simulink model "ABS_CHO"  (R2023a)
settings: Solver=ode45  StartTime=0  StopTime=15  FixedStep=0.001  RelTol=1e-3  AbsTol=1e-6
libraries: simulink x19, dspsigops x7, Solver_SF x1
(part 2 of 2)

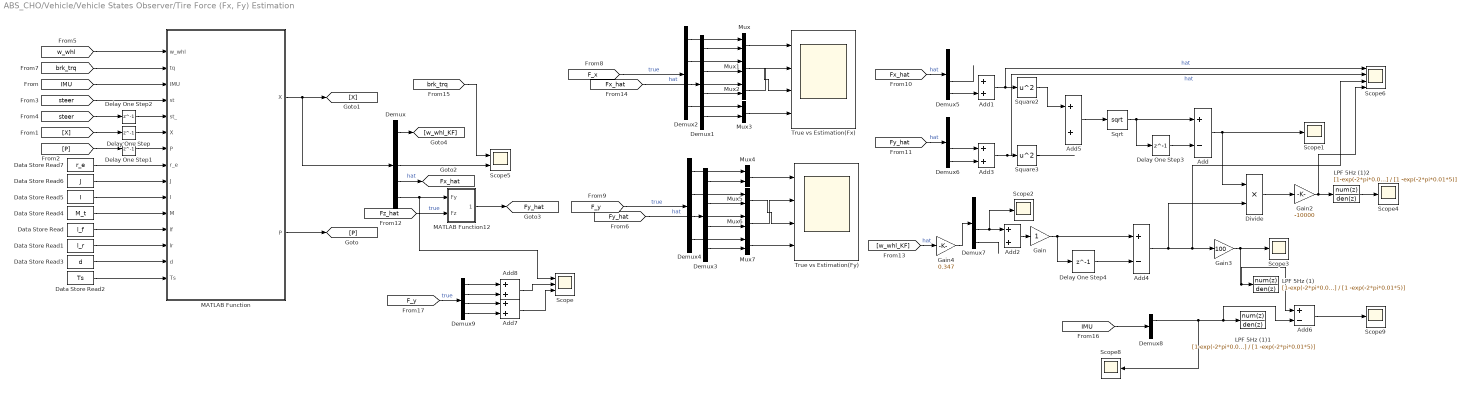
== system ABS_CHO/Vehicle/Vehicle States Observer/Tire Force (Fx, Fy) Estimation ==
  Add : Sum  Inputs=+-
  Add{1..3,5,7..8} (6 alike) : Sum
  Add4 : Sum  Inputs=+-
  Add6 : Sum  Inputs=+-
  Data Store Read : DataStoreRead  DataStoreName=l_f  IndexOptions=Index vector (dialog)  Indices=1  OutputSizes=1
  Data Store Read1 : DataStoreRead  DataStoreName=l_r  IndexOptions=Index vector (dialog)  Indices=1  OutputSizes=1
  Data Store Read2 : DataStoreRead  DataStoreName=Ts  IndexOptions=Index vector (dialog)  Indices=1  OutputSizes=1
  Data Store Read3 : DataStoreRead  DataStoreName=d  IndexOptions=Index vector (dialog)  Indices=1  OutputSizes=1
  Data Store Read4 : DataStoreRead  DataStoreName=M_t  IndexOptions=Index vector (dialog)  Indices=1  OutputSizes=1
  Data Store Read5 : DataStoreRead  DataStoreName=I  IndexOptions=Index vector (dialog)  Indices=1  OutputSizes=1
  Data Store Read6 : DataStoreRead  DataStoreName=J  IndexOptions=Index vector (dialog)  Indices=1  OutputSizes=1
  Data Store Read7 : DataStoreRead  DataStoreName=r_e  IndexOptions=Index vector (dialog)  Indices=1  OutputSizes=1
  Delay One Step : Delay  DelayLength=1  InitialCondition=[80 80 80 80 0 0 0 0 0 0 0 0]'  SampleTime=0.01
  Delay One Step1 : Delay  DelayLength=1  InitialCondition=diag([80 80 80 80 0 0 0 0 0 0 0 0])  SampleTime=0.01
  Delay One Step2 : Delay  DelayLength=1  InitialCondition=[0 0 0 0]'  SampleTime=0.01
  Delay One Step3 : Delay  DelayLength=1
  Delay One Step4 : Delay  DelayLength=1  InitialCondition=27.78
  Demux : Demux  Outputs=[4 1 1 4 2]
  Demux{1..7,9} (8 alike) : Demux
  Demux8 : Demux  Outputs=3
  Divide : Product  Inputs=**
  Gain : Gain
  Gain2 : Gain  Gain=-10000
  Gain3 : Gain  Gain=100
  Gain4 : Gain  Gain=0.347
  LPF 5Hz (1) : DiscreteFilter  Numerator=[1-exp(-2*pi*0.01*5)]  Denominator=[1 -exp(-2*pi*0.01*5)]  SampleTime=0.01
  LPF 5Hz (1)1 : DiscreteFilter  Numerator=[1-exp(-2*pi*0.01*5)]  Denominator=[1 -exp(-2*pi*0.01*5)]  SampleTime=0.01
  LPF 5Hz (1)2 : DiscreteFilter  Numerator=[1-exp(-2*pi*0.01*5)]  Denominator=[1 -exp(-2*pi*0.01*5)]  SampleTime=0.01
  MATLAB Function : MATLAB Function  TreatAsAtomicUnit=on
  MATLAB Function12 : MATLAB Function  TreatAsAtomicUnit=on
  Mux{,1..7} (8 alike) : Mux  Inputs=2
  Scope : Scope  NumInputPorts=3
  Scope{1..4,8..9} (6 alike) : Scope
  Scope5 : Scope  NumInputPorts=2
  Scope6 : Scope  NumInputPorts=4
  Sqrt : Sqrt
  Square2 : Math  Operator=square
  Square3 : Math  Operator=square
  True vs Estimation(Fx) : Scope  NumInputPorts=4
  True vs Estimation(Fy) : Scope  NumInputPorts=4
  tag scope: Fx_hat=global, Fy_hat=global
  wires:
  Data Store Read/1 -> MATLAB Function/12(lf)
  Data Store Read1/1 -> MATLAB Function/13(lr)
  Data Store Read2/1 -> MATLAB Function/15(Ts)
  Data Store Read3/1 -> MATLAB Function/14(d)
  Data Store Read4/1 -> MATLAB Function/11(M)
  Data Store Read5/1 -> MATLAB Function/10(I)
  Data Store Read6/1 -> MATLAB Function/9(J)
  Data Store Read7/1 -> MATLAB Function/8(r_e)
  MATLAB Function/2(P) -> [P]
  MATLAB Function/1(X) -> Demux/1, [X]
  [X] -> Delay One Step/1
  Delay One Step/1 -> MATLAB Function/6("X ")
  [P] -> Delay One Step1/1
  Delay One Step1/1 -> MATLAB Function/7("P ")
  [steer] -> MATLAB Function/4(st)
  [steer] -> Delay One Step2/1
  Delay One Step2/1 -> MATLAB Function/5(st_)
  [w_whl] -> MATLAB Function/1(w_whl)
  Mux2/1 -> True vs Estimation(Fx)/2
  Mux3/1 -> True vs Estimation(Fx)/4
  Demux1/3 -> Mux2/2
  Mux/1 -> True vs Estimation(Fx)/1
  [Fx_hat] -> Demux1/1  "hat"
  Demux1/4 -> Mux3/2
  Demux2/4 -> Mux3/1
  Demux1/2 -> Mux1/2
  Demux1/1 -> Mux/2
  Demux2/1 -> Mux/1
  Demux2/3 -> Mux2/1
  Mux1/1 -> True vs Estimation(Fx)/3
  Demux2/2 -> Mux1/1
  [F_x] -> Demux2/1  "true"
  [IMU] -> MATLAB Function/3(IMU)
  [brk_trq] -> MATLAB Function/2(tq)
  [Fz_hat] -> MATLAB Function12/2(Fz)  "true"
  Demux/4 -> [Fx_hat]  "hat"
  Demux/5 -> Scope/1, MATLAB Function12/1(Fy)
  MATLAB Function12/1(Fyhat) -> [Fy_hat]
  Demux4/1 -> Mux4/1
  Demux4/2 -> Mux5/1
  Demux3/4 -> Mux7/2
  Demux3/2 -> Mux5/2
  Demux3/1 -> Mux4/2
  Demux4/3 -> Mux6/1
  Demux4/4 -> Mux7/1
  Mux7/1 -> True vs Estimation(Fy)/4
  Mux6/1 -> True vs Estimation(Fy)/2
  Demux3/3 -> Mux6/2
  [F_y] -> Demux4/1  "true"
  Mux5/1 -> True vs Estimation(Fy)/3
  Mux4/1 -> True vs Estimation(Fy)/1
  [Fy_hat] -> Demux3/1  "hat"
  [Fx_hat] -> Demux5/1  "hat"
  Add1/1 -> Scope6/1, Square2/1  "hat"
  Demux5/3 -> ?
  Demux5/4 -> Add1/2
  Demux6/3 -> Add3/1
  [Fy_hat] -> Demux6/1  "hat"
  Add3/1 -> Scope6/2, Square3/1  "hat"
  Demux6/4 -> Add3/2
  Square2/1 -> Add5/1
  Square3/1 -> ?
  Delay One Step3/1 -> Add/2
  Add/1 -> Divide/1, Scope1/1
  Add5/1 -> Sqrt/1
  Sqrt/1 -> Delay One Step3/1, Add/1
  [w_whl_KF] -> Gain4/1  "hat"
  Demux7/3 -> Scope2/1, Add2/1
  Demux7/4 -> ?
  Add2/1 -> Gain/1
  Gain/1 -> Delay One Step4/1, Add4/1
  Delay One Step4/1 -> Add4/2
  Add4/1 -> Divide/2, Gain3/1, Scope6/3
  Divide/1 -> Gain2/1
  Demux/3 -> Scope5/2
  [brk_trq] -> Scope5/1
  Gain3/1 -> Add6/1, LPF 5Hz (1)/1, Scope3/1
  Demux/1 -> [w_whl_KF]
  [IMU] -> Demux8/1
  Demux8/1 -> Scope8/1, Add6/2, LPF 5Hz (1)1/1
  Add6/1 -> Scope9/1
  Gain2/1 -> LPF 5Hz (1)2/1, Scope6/4
  LPF 5Hz (1)2/1 -> Scope4/1
  Gain4/1 -> Demux7/1
  [F_y] -> Demux9/1  "true"
  Demux9/4 -> Add7/2
  Demux9/3 -> Add7/1
  Demux9/1 -> Add8/1
  Demux9/2 -> Add8/2
  Add8/1 -> Scope/2
  Add7/1 -> Scope/3

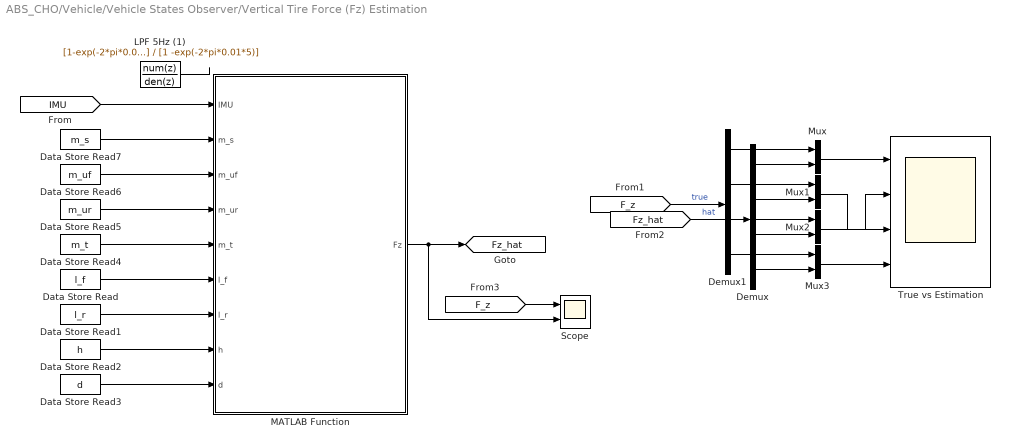
== system ABS_CHO/Vehicle/Vehicle States Observer/Vertical Tire Force (Fz) Estimation ==
  Data Store Read : DataStoreRead  DataStoreName=l_f  IndexOptions=Index vector (dialog)  Indices=1  OutputSizes=1
  Data Store Read1 : DataStoreRead  DataStoreName=l_r  IndexOptions=Index vector (dialog)  Indices=1  OutputSizes=1
  Data Store Read2 : DataStoreRead  DataStoreName=h  IndexOptions=Index vector (dialog)  Indices=1  OutputSizes=1
  Data Store Read3 : DataStoreRead  DataStoreName=d  IndexOptions=Index vector (dialog)  Indices=1  OutputSizes=1
  Data Store Read4 : DataStoreRead  DataStoreName=m_t  IndexOptions=Index vector (dialog)  Indices=1  OutputSizes=1
  Data Store Read5 : DataStoreRead  DataStoreName=m_ur  IndexOptions=Index vector (dialog)  Indices=1  OutputSizes=1
  Data Store Read6 : DataStoreRead  DataStoreName=m_uf  IndexOptions=Index vector (dialog)  Indices=1  OutputSizes=1
  Data Store Read7 : DataStoreRead  DataStoreName=m_s  IndexOptions=Index vector (dialog)  Indices=1  OutputSizes=1
  Demux : Demux
  Demux1 : Demux
  LPF 5Hz (1) : DiscreteFilter  Numerator=[1-exp(-2*pi*0.01*5)]  Denominator=[1 -exp(-2*pi*0.01*5)]  SampleTime=0.01
  MATLAB Function : MATLAB Function  TreatAsAtomicUnit=on
  Mux{,1..3} (4 alike) : Mux  Inputs=2
  Scope : Scope  NumInputPorts=2
  True vs Estimation : Scope  NumInputPorts=4
  tag scope: Fz_hat=global
  wires:
  Data Store Read/1 -> MATLAB Function/6(l_f)
  Data Store Read1/1 -> MATLAB Function/7(l_r)
  Data Store Read2/1 -> MATLAB Function/8(h)
  Data Store Read3/1 -> MATLAB Function/9(d)
  Data Store Read4/1 -> MATLAB Function/5(m_t)
  Data Store Read5/1 -> MATLAB Function/4(m_ur)
  Data Store Read6/1 -> MATLAB Function/3(m_uf)
  Data Store Read7/1 -> MATLAB Function/2(m_s)
  [IMU] -> MATLAB Function/1(IMU)
  MATLAB Function/1(Fz) -> Scope/2, [Fz_hat]
  [F_z] -> Scope/1
  [Fz_hat] -> Demux/1  "hat"
  [F_z] -> Demux1/1  "true"
  Demux1/1 -> Mux/1
  Demux/1 -> Mux/2
  Demux1/2 -> Mux1/1
  Demux/2 -> Mux1/2
  Demux1/3 -> Mux2/1
  Demux/3 -> Mux2/2
  Demux1/4 -> Mux3/1
  Demux/4 -> Mux3/2
  Mux/1 -> True vs Estimation/1
  Mux1/1 -> True vs Estimation/3
  Mux3/1 -> True vs Estimation/4
  Mux2/1 -> True vs Estimation/2
  LPF 5Hz (1)/1 -> ?

== stateflow chart ABS_CHO/ABS_FR/Chart ==
  state ABS_On
    state Phase1
      entry,during:
      phase = 1;
    state Phase2
      entry,during:
      phase = 2;
    state Phase3
      entry,during:
      phase = 3;
    state Phase4
      entry,during:
      phase = 4;
    state Phase5
      entry,during:
      phase = 5;
    state Phase6
      entry,during:
      phase = 6;
    state Phase7
      entry,during:
      phase = 7;
    state Phase8
      entry,during:
      phase = 8;
    (default) -> Phase1
    Phase1 -> Phase2 : [(a_whl<a_whl_thrs1)]
    Phase2 -> Phase3 : [(v_whl<v_whl_thrs)]
    Phase3 -> Phase4 : [(a_whl>a_whl_thrs1)]
    (junction 81) -> Phase4
    (junction 79) -> (junction 81)
    Phase4 -> Phase5 : [(a_whl>a_whl_thrs2)]
    Phase5 -> Phase6 : [(a_whl<a_whl_thrs2)]
    Phase6 -> Phase7 : [(a_whl<a_whl_thrs3)]
    Phase7 -> Phase8 : [(a_whl<a_whl_thrs1)]
    Phase8 -> (junction 79) : [(a_whl>a_whl_thrs1)]
  state ABS_Off
    phase = 0;
  (default) -> ABS_Off
  ABS_Off -> ABS_On : [(P_cmd > P_cmd_min)&(v_car > 2)]
  (junction 96) -> ABS_Off
  ABS_On -> (junction 96) : [(P_cmd < P_cmd_min)|(v_car < 2)]
  data: a_whl input; phase output; v_whl input; v_car input; P_cmd input; P_cmd_min input; a_whl_thrs1 input; a_whl_thrs2 input; a_whl_thrs3 input; v_whl_thrs input

== stateflow chart ABS_CHO/ABS_FL/Chart ==
  state ABS_On
    state Phase1
      entry,during:
      phase = 1;
    state Phase2
      entry,during:
      phase = 2;
    state Phase3
      entry,during:
      phase = 3;
    state Phase4
      entry,during:
      phase = 4;
    state Phase5
      entry,during:
      phase = 5;
    state Phase6
      entry,during:
      phase = 6;
    state Phase7
      entry,during:
      phase = 7;
    state Phase8
      entry,during:
      phase = 8;
    (default) -> Phase1
    Phase1 -> Phase2 : [(a_whl<a_whl_thrs1)]
    Phase2 -> Phase3 : [(v_whl<v_whl_thrs)]
    Phase3 -> Phase4 : [(a_whl>a_whl_thrs1)]
    (junction 81) -> Phase4
    (junction 79) -> (junction 81)
    Phase4 -> Phase5 : [(a_whl>a_whl_thrs2)]
    Phase5 -> Phase6 : [(a_whl<a_whl_thrs2)]
    Phase6 -> Phase7 : [(a_whl<a_whl_thrs3)]
    Phase7 -> Phase8 : [(a_whl<a_whl_thrs1)]
    Phase8 -> (junction 79) : [(a_whl>a_whl_thrs1)]
  state ABS_Off
    phase = 0;
  (default) -> ABS_Off
  ABS_Off -> ABS_On : [(P_cmd > P_cmd_min)&(v_car > 2)]
  (junction 96) -> ABS_Off
  ABS_On -> (junction 96) : [(P_cmd < P_cmd_min)|(v_car < 2)]
  data: a_whl input; phase output; v_whl input; v_car input; P_cmd input; P_cmd_min input; a_whl_thrs1 input; a_whl_thrs2 input; a_whl_thrs3 input; v_whl_thrs input

== stateflow chart ABS_CHO/ABS_RR/Chart ==
  state ABS_On
    state Phase1
      entry,during:
      phase = 1;
    state Phase2
      entry,during:
      phase = 2;
    state Phase3
      entry,during:
      phase = 3;
    state Phase4
      entry,during:
      phase = 4;
    state Phase5
      entry,during:
      phase = 5;
    state Phase6
      entry,during:
      phase = 6;
    state Phase7
      entry,during:
      phase = 7;
    state Phase8
      entry,during:
      phase = 8;
    (default) -> Phase1
    Phase1 -> Phase2 : [(a_whl<a_whl_thrs1)]
    Phase2 -> Phase3 : [(v_whl<v_whl_thrs)]
    Phase3 -> Phase4 : [(a_whl>a_whl_thrs1)]
    (junction 81) -> Phase4
    (junction 79) -> (junction 81)
    Phase4 -> Phase5 : [(a_whl>a_whl_thrs2)]
    Phase5 -> Phase6 : [(a_whl<a_whl_thrs2)]
    Phase6 -> Phase7 : [(a_whl<a_whl_thrs3)]
    Phase7 -> Phase8 : [(a_whl<a_whl_thrs1)]
    Phase8 -> (junction 79) : [(a_whl>a_whl_thrs1)]
  state ABS_Off
    phase = 0;
  (default) -> ABS_Off
  ABS_Off -> ABS_On : [(P_cmd > P_cmd_min)&(v_car > 2)]
  (junction 96) -> ABS_Off
  ABS_On -> (junction 96) : [(P_cmd < P_cmd_min)|(v_car < 2)]
  data: a_whl input; phase output; v_whl input; v_car input; P_cmd input; P_cmd_min input; a_whl_thrs1 input; a_whl_thrs2 input; a_whl_thrs3 input; v_whl_thrs input

== stateflow chart ABS_CHO/ABS_RL/Chart ==
  state ABS_On
    state Phase1
      entry,during:
      phase = 1;
    state Phase2
      entry,during:
      phase = 2;
    state Phase3
      entry,during:
      phase = 3;
    state Phase4
      entry,during:
      phase = 4;
    state Phase5
      entry,during:
      phase = 5;
    state Phase6
      entry,during:
      phase = 6;
    state Phase7
      entry,during:
      phase = 7;
    state Phase8
      entry,during:
      phase = 8;
    (default) -> Phase1
    Phase1 -> Phase2 : [(a_whl<a_whl_thrs1)]
    Phase2 -> Phase3 : [(v_whl<v_whl_thrs)]
    Phase3 -> Phase4 : [(a_whl>a_whl_thrs1)]
    (junction 81) -> Phase4
    (junction 79) -> (junction 81)
    Phase4 -> Phase5 : [(a_whl>a_whl_thrs2)]
    Phase5 -> Phase6 : [(a_whl<a_whl_thrs2)]
    Phase6 -> Phase7 : [(a_whl<a_whl_thrs3)]
    Phase7 -> Phase8 : [(a_whl<a_whl_thrs1)]
    Phase8 -> (junction 79) : [(a_whl>a_whl_thrs1)]
  state ABS_Off
    phase = 0;
  (default) -> ABS_Off
  ABS_Off -> ABS_On : [(P_cmd > P_cmd_min)&(v_car > 2)]
  (junction 96) -> ABS_Off
  ABS_On -> (junction 96) : [(P_cmd < P_cmd_min)|(v_car < 2)]
  data: a_whl input; phase output; v_whl input; v_car input; P_cmd input; P_cmd_min input; a_whl_thrs1 input; a_whl_thrs2 input; a_whl_thrs3 input; v_whl_thrs input

== matlab function ABS_CHO/Vehicle/Vehicle States Observer/Vertical Tire Force (Fz) Estimation/MATLAB Function ==
  data: IMU input; m_s input; m_uf input; m_ur input; m_t input; l_f input; l_r input; h input; d input; Fz output
function Fz = fcn(IMU, m_s, m_uf, m_ur, m_t, l_f, l_r, h, d)

a = [9.8 IMU(1) IMU(2)]';

L = l_f+l_r;
Mz = [l_r/(2*L)*m_s+1/2*m_uf+m_t -h/(2*L)*m_s -h/(4*d)*m_s;
     l_r/(2*L)*m_s+1/2*m_uf+m_t -h/(2*L)*m_s h/(4*d)*m_s;
     l_f/(2*L)*m_s+1/2*m_ur+m_t h/(2*L)*m_s -h/(4*d)*m_s;
     l_f/(2*L)*m_s+1/2*m_ur+m_t h/(2*L)*m_s h/(4*d)*m_s];

Fz = Mz*a;

== matlab function ABS_CHO/Vehicle/Vehicle States Observer/Tire Force (Fx, Fy) Estimation/MATLAB Function ==
  data: w_whl input; tq input; IMU input; st input; st_ input; X input; P input; X output; P output; r_e input; J input; I input; M input; lf input; lr input; d input; Ts input
function [X,P]  = fcn(w_whl,tq,IMU,st,st_,X,P,r_e,J,I,M,lf,lr,d,Ts)

delta_ = (st_(1)+st_(2))/2;
delta = (st(1)+st(2))/2;

%X = [w_FL w_FR w_RL w_RR r tq_h Fx_FL Fx_FR Fx_RL Fx_RR Fy_F Fy_R]
Q = diag([0.001 0.001 0.00028 0.00028 0.000001 100 1000 1000 50 50 1000 1000]);

Z = [w_whl(1) w_whl(2) w_whl(3) w_whl(4) IMU(3) IMU(1) IMU(2)]';
R = diag([0.00028 0.00028 0.00028 0.00028 0.000001 0.001 0.001]);

U = [0 -tq(3)]';

F = eye(12) + Ts*...
    [0 0 0 0 0 -1/J r_e/J 0 0 0 0 0;
     0 0 0 0 0 -1/J 0 r_e/J 0 0 0 0;
     0 0 0 0 0 0 0 0 r_e/J 0 0 0;
     0 0 0 0 0 0 0 0 0 r_e/J 0 0;
     0 0 0 0 0 0 -lf/I*sin(st_(1))+d/I*cos(st_(1)) -lf/I*sin(st_(2))-d/I*cos(st_(2)) d/I -d/I lf/I*cos(delta_) -lr/I;
     zeros(7,12)];

G = Ts/J*[-1 0; -1 0; 0 -1; 0 -1;zeros(8,2)];

H = [eye(5) zeros(5,7);
     zeros(1,6) -cos(st(1))/M -cos(st(2))/M -1/M -1/M -sin(delta)/M 0;
     zeros(1,6) -sin(st(1))/M -sin(st(2))/M 0 0 cos(delta)/M 1/M];

Xm = F*X + G*U;
Pm = F*P*F' + Q;
K = Pm*H'/(H*Pm*H'+R);
X = Xm + K*(Z-H*Xm);
P = (eye(12)-K*H)*Pm;

end

== matlab function ABS_CHO/Vehicle/Vehicle States Observer/Rear Wheel Torque Control/MATLAB Function ==
  data: ABS_flag output; r_e input; sgn output; w input; wdot input; V_hat input; IMU input; ABS_flag input; case_flag input; sgn_ input; Fx input; Fxdot input; Fy input; Fz input; case_flag output; mu_max output; mu_max input; brk_stat input; a output
function [ABS_flag,sgn,case_flag,mu_max,a]  = fcn(r_e,w,wdot,V_hat,IMU,ABS_flag,case_flag,sgn_,Fx,Fxdot,Fy,Fz,mu_max,brk_stat)

% Rear Left
w = w(3); wdot = wdot(3); V_hat = V_hat(3);
Fx = Fx(3); Fxdot = Fxdot(3); Fy = Fy(3); Fz = Fz(3);
% 휠 슬립율이 변화중이어야만 sgn 갱신
if abs(r_e*wdot-1*IMU(1)) > 10 && brk_stat == 1
    sgn = -Fxdot*(r_e*wdot-1*IMU(1));
else
    sgn = sgn_;
end

if sgn >= 0
    sgn = 1;
else
    sgn = -1;
end

%case 1
if sgn == 1 && r_e*w < 0.7*V_hat && case_flag ~=1
    ABS_flag = 1;
    case_flag = 1;
    mu_max = sqrt(Fx^2+Fy^2)/Fz;

elseif sgn ~= sgn_
    ABS_flag = 1;
    case_flag = 2;
    mu_max = sqrt(Fx^2+Fy^2)/Fz;
else
end
a = r_e*wdot-0.9*IMU(1);

== matlab function ABS_CHO/Vehicle/Vehicle States Observer/Rear Wheel Torque Control/MATLAB Function1 ==
  data: ABS_flag output; r_e input; sgn output; w input; wdot input; V_hat input; IMU input; ABS_flag input; case_flag input; sgn_ input; Fx input; Fxdot input; Fy input; Fz input; case_flag output; mu_max output; mu_max input; brk_stat input; a output
function [ABS_flag,sgn,case_flag,mu_max,a]  = fcn(r_e,w,wdot,V_hat,IMU,ABS_flag,case_flag,sgn_,Fx,Fxdot,Fy,Fz,mu_max,brk_stat)

% Rear Right
w = w(4); wdot = wdot(4); V_hat = V_hat(4);
Fx = Fx(4); Fxdot = Fxdot(4); Fy = Fy(4); Fz = Fz(4);
% 휠 슬립율이 변화중이어야만 sgn 갱신
if abs(r_e*wdot-1*IMU(1)) > 10 && brk_stat == 1
    sgn = -Fxdot*(r_e*wdot-1*IMU(1));
else
    sgn = sgn_;
end

if sgn >= 0
    sgn = 1;
else
    sgn = -1;
end

%case 1
if sgn == 1 && r_e*w < 0.7*V_hat && case_flag ~=1
    ABS_flag = 1;
    case_flag = 1;
    mu_max = sqrt(Fx^2+Fy^2)/Fz;

elseif sgn ~= sgn_
    ABS_flag = 1;
    case_flag = 2;
    mu_max = sqrt(Fx^2+Fy^2)/Fz;
else
end
a = r_e*wdot-IMU(1);

== matlab function ABS_CHO/Vehicle/Vehicle States Observer/Rear Wheel Torque Control/MATLAB Function2 ==
  data: case_flag input; sgn input; tq_cmd input; mu_max input; Fx input; Fy input; Fz input; r_e input; tq_out output; J input
function tq_out = fcn(case_flag,sgn,tq_cmd,mu_max,Fx,Fy,Fz,r_e,J)

% Rear Left
Fx = Fx(3); Fy = Fy(3); Fz = Fz(3);
if case_flag == 1
    tq_out = r_e*sqrt(max((mu_max*Fz)^2-Fy^2,0)) + J*mu_max*9.8/r_e;
elseif case_flag == 2
    tq_out = r_e*Fx + J/r_e*mu_max*9.8 + 70*sgn;
else
    tq_out = tq_cmd;
end

== matlab function ABS_CHO/Vehicle/Vehicle States Observer/Rear Wheel Torque Control/MATLAB Function3 ==
  data: case_flag input; sgn input; tq_cmd input; mu_max input; Fx input; Fy input; Fz input; r_e input; tq_out output; J input
function tq_out = fcn(case_flag,sgn,tq_cmd,mu_max,Fx,Fy,Fz,r_e,J)

% Rear Left
Fx = Fx(4); Fy = Fy(4); Fz = Fz(4);
if case_flag == 1
    tq_out = r_e*sqrt(max((mu_max*Fz)^2-Fy^2,0)) + J*mu_max*9.8/r_e;
elseif case_flag == 2
    tq_out = r_e*Fx + J/r_e*mu_max*9.8 + 70*sgn;
else
    tq_out = tq_cmd;
end

== matlab function ABS_CHO/Vehicle/Vehicle States Observer/Rear Wheel Torque Control/MATLAB Function4 ==
  data: u input; phase output; thrs input; phase input; sgn input; sgn output
function [phase,sgn] = fcn(u,thrs,phase,sgn)
for i = 1:4
    if abs(u(i)) > thrs
        if u(i) > 0
            phase(i) = 1; sgn(i) = 1;
        else
            phase(i) = -1; sgn(i) = -1;
        end
    else
        phase(i) = 0;
        % if phase(i) == 1
        %     sgn(i) = -1; phase(i) = 0;
        % elseif phase(i) == -1
        %     sgn(i) = 1; phase(i) = 0;
        % else
        % 
        % end
    end
end

== matlab function ABS_CHO/Vehicle/Vehicle States Observer/Rear Wheel Torque Control/MATLAB Function5 ==
  data: r_e input; u input; IMU input; phase output; thrs input; phase input; sgn input; sgn output
function [phase,sgn] = fcn(r_e,u,IMU,thrs,phase,sgn)
u = r_e*u - 0.9*IMU(1);
for i = 1:4
    if abs(u(i)) > thrs
        if u(i) > 0
            phase(i) = 1; sgn(i) = 1;
        else
            phase(i) = -1; sgn(i) = -1;
        end
    else        
        if phase(i) == 1
            sgn(i) = -1; phase(i) = 0;
        elseif phase(i) == -1
            sgn(i) = 1; phase(i) = 0;
        else

        end
    end
end

== matlab function ABS_CHO/Vehicle/Vehicle States Observer/Rear Wheel Torque Control/MATLAB Function6 ==
  data: ABS_flag output; sgn output; phasewd input; phaseFxd input; ABS_flag input; sgn_ input; Fx input; Fy input; Fz input; mu_max output; mu_max input; brk_stat input; zerophase input; zerophase output
function [ABS_flag,sgn,mu_max,zerophase]  = fcn(phasewd,phaseFxd,ABS_flag,sgn_,Fx,Fy,Fz,mu_max,brk_stat,zerophase)

% Rear Left
wd = phasewd(3); Fx = Fx(3); Fxd = phaseFxd(3); Fy = Fy(3); Fz = Fz(3);
if brk_stat == 1

    if wd == 0
        
        sgn = 0;
    else
        sgn = wd*Fxd;
    end

    if sgn-sgn_ < 0
        ABS_flag = 1;
    end
    if abs(sgn-sgn_) > 0 && ABS_flag == 1
        mu_max = sqrt(Fx^2+Fy^2)/Fz;
    end
else
    sgn = sgn_;
end

== matlab function ABS_CHO/Vehicle/Vehicle States Observer/Rear Wheel Torque Control/MATLAB Function7 ==
  data: u input; phase output; thrs input; phase input
function phase  = fcn(u,thrs,phase)
for i = 1:4
    if u(i) > thrs
        phase(i) = 1;
    elseif u(i) < -thrs
        phase(i) = -1;
    else
        phase(i) = 0;
    end
end

== matlab function ABS_CHO/Vehicle/Vehicle States Observer/Tire Force (Fx, Fy) Estimation/MATLAB Function12 ==
  data: Fy input; Fz input; Fyhat output
function Fyhat = fcn(Fy, Fz)

kf = Fz(1)/Fz(2);
kr = Fz(3)/Fz(4);

Fylf = kf/(1+kf)*Fy(1);
Fyrf = 1/(1+kf)*Fy(1);
Fylr = kr/(1+kr)*Fy(2);
Fyrr = 1/(1+kr)*Fy(2);

Fyhat = [Fylf Fyrf Fylr Fyrr]';

== matlab function ABS_CHO/Vehicle/Vehicle States Observer/Rear Wheel Torque Control/MATLAB Function8 ==
  data: r_e input; u input; IMU input; phase output; thrs input; phase input
function phase  = fcn(r_e,u,IMU,thrs,phase)
u = r_e*u -IMU(1);
for i = 1:4
    if u(i) > thrs
        phase(i) = -1;
    elseif u(i) < -thrs
        phase(i) = 1;
    else
        phase(i) = 0;
    end
end

== matlab function ABS_CHO/Vehicle/Vehicle States Observer/Rear Wheel Torque Control/MATLAB Function9 ==
  data: ABS_flag output; sgn output; phasewd input; phaseFxd input; ABS_flag input; sgn_ input; Fx input; Fy input; Fz input; mu_max output; mu_max input; brk_stat input; zerophase input; zerophase output
function [ABS_flag,sgn,mu_max,zerophase]  = fcn(phasewd,phaseFxd,ABS_flag,sgn_,Fx,Fy,Fz,mu_max,brk_stat,zerophase)

% Rear Left
wd = phasewd(4); Fx = Fx(4); Fxd = phaseFxd(4); Fy = Fy(4); Fz = Fz(4);
if brk_stat == 1

    if wd == 0
        sgn = sgn_;
    else
        sgn = wd*Fxd;
    end

    if sgn-sgn_ < 0
        ABS_flag = 1;
    end
    if abs(sgn-sgn_) > 0 && ABS_flag == 1
        mu_max = sqrt(Fx^2+Fy^2)/Fz;
    end
else
    sgn = sgn_;
end

== matlab function ABS_CHO/Vehicle/Vehicle States Observer/Rear Wheel Torque Control/MATLAB Function10 ==
  data: ABS_flag input; sgn input; tq_cmd input; mu_max input; Fx input; r_e input; tq_out output; J input
function tq_out = fcn(ABS_flag,sgn,tq_cmd,mu_max,Fx,r_e,J)

% Rear Left
Fx = Fx(3);

if ABS_flag == 1
    tq_out = r_e*Fx + J/r_e*mu_max*9.8 + 50*sgn;
else
    tq_out = tq_cmd;
end

== matlab function ABS_CHO/Vehicle/Vehicle States Observer/Rear Wheel Torque Control/MATLAB Function11 ==
  data: ABS_flag input; sgn input; tq_cmd input; mu_max input; Fx input; r_e input; tq_out output; J input
function tq_out = fcn(ABS_flag,sgn,tq_cmd,mu_max,Fx,r_e,J)

% Rear Left
Fx = Fx(3);

if ABS_flag == 1
    tq_out = r_e*Fx + J/r_e*mu_max*9.8 + 50*sgn;
else
    tq_out = tq_cmd;
end

== stateflow chart ABS_CHO/Vehicle/Vehicle States Observer/Rear Wheel Torque Control/Chart2 ==
  state Phase2
    entry, during:
    ABS_flag = 1;
    sgn = -1;
    phase = 2;
  state Phase3
    entry, during:
    ABS_flag = 1;
    sgn = -1;
    phase = 3;
  state ABS_off
    entry, during:
    ABS_flag = 0;
    sgn = 0;
    phase = 0;
  state Phase1
    entry, during:
    ABS_flag = 1;
    sgn = 0;
    phase = 1;
    mu_max = mu;
  state Phase4
    entry, during:
    ABS_flag = 1;
    sgn = 1;
    phase = 4;
  Phase2 -> Phase3 : [(Fxd == 1)&(wd == -1)]
  Phase1 -> Phase2 [order 3] : [(wd > -1)&(Fxd == -1)]
  Phase1 -> Phase3 [order 2] : [(wd == -1)&(Fxd == 1)]
  (default) -> ABS_off
  ABS_off -> Phase1 : [(Fxd-Fxd_ < 0)&(wd == 1)]
  Phase3 -> Phase1 [order 2] : [(wd == -1)&(Fxd == 0)]
  Phase3 -> (junction 25) [order 1]
  Phase4 -> Phase1 : [(Fxd == 0)&(wd == 1)]
  Phase1 -> Phase4 [order 1] : [(wd == -1)&(Fxd == -1)]
  (junction 25) -> Phase4 : [(Fxd == -1)]
  data: Fxd input; wd input; sgn output; phase output; ABS_flag output; mu input; mu_max output; Fxd_ input

== stateflow chart ABS_CHO/Vehicle/Vehicle States Observer/Rear Wheel Torque Control/Chart1 ==
  state Phase2
    entry, during:
    ABS_flag = 1;
    sgn = -1;
    phase = 2;
  state Phase3
    entry, during:
    ABS_flag = 1;
    sgn = -1;
    phase = 3;
  state ABS_off
    entry, during:
    ABS_flag = 0;
    sgn = 0;
    phase = 0;
  state Phase1
    entry, during:
    ABS_flag = 1;
    sgn = 0;
    phase = 1;
    mu_max = mu;
  state Phase4
    entry, during:
    ABS_flag = 1;
    sgn = 1;
    phase = 4;
  Phase2 -> Phase3 : [(Fxd == 1)&(wd == -1)]
  Phase1 -> Phase2 [order 3] : [(wd > -1)&(Fxd == -1)]
  Phase1 -> Phase3 [order 2] : [(wd == -1)&(Fxd == 1)]
  (default) -> ABS_off
  ABS_off -> Phase1 : [(Fxd-Fxd_ < 0)&(wd == 1)]
  Phase3 -> Phase1 [order 2] : [(wd == -1)&(Fxd == 0)]
  Phase3 -> (junction 25) [order 1]
  Phase4 -> Phase1 : [(Fxd == 0)&(wd == 1)]
  Phase1 -> Phase4 [order 1] : [(wd == -1)&(Fxd == -1)]
  (junction 25) -> Phase4 : [(Fxd == -1)]
  data: Fxd input; wd input; sgn output; phase output; ABS_flag output; mu input; mu_max output; Fxd_ input
